simulink library "MantaFSController_cl"  (R2020a)
settings: Solver=VariableStepAuto  StartTime=0.0  StopTime=10.0  RelTol=1e-3
undefined symbols (not defined in the file or in its folder): a, env, FLIGHTCONTROLLER, fltCtrl, initializeBussesFromBlock, pthCtrl1, pthCtrl2, slfCtrl, thr, vhcl, wnch
libraries: simulink x21, angleBtw2Vecs_ul x9, pathGeometry_ul x6, filteredPIDController_ul x5, ctrlAllocMatrix_cl x4, tanFrameProjection_ul x4, vectorNormalizer_ul x4, velocityAngle_ul x4, filteredPIDControllerAWGS_ul x3, eulAng2RotMat_ul x3, vrlib x3, alphaBeta_ul x3
(part 1 of 3)
settings Model: Creator=jldanie5  LastModifiedBy=JohnJr
settings DataIOCC: ReturnWorkspaceOutputs=off
settings DebuggingCC: ArithmeticOperatorsInVariantConditions=warning
settings SFSimCC: CustomCodeUndefinedFunction=UseInterfaceOnly

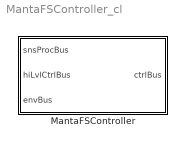
== system MantaFSController_cl ==
  MantaFSController : Subsystem  LoadFcn=initializeBussesFromBlock(gcb)  InitFcn=initializeBussesFromBlock(gcb)  StartFcn=initializeBussesFromBlock(gcb)  VariantControl=strcmpi(FLIGHTCONTROLLER,'MantaFSController')  mask{initPosForInitSStar=vhcl.initPosVecGnd.Value, fluidDensity=env.water.density.Value, LaRCtrl=fltCtrl, aeroStruct=vhcl.struct('OCT.aeroSurf'), LaRThr=thr.tether1, LaRWnch=wnch.winch1}
      mask prompts: initPosForInitSStar "Initial Position"; fluidDensity "Fluid Density"; LaRCtrl "Controller"; aeroStruct "Aerodynamic Structure"; LaRThr "Tether"; LaRWnch "Winch"
      settings: MinAlgLoopOccurrences=on
      mask DialogControl Container3 Prompt: Course Follow Params
      mask DialogControl Container4 Prompt: Setpoint To Output Params

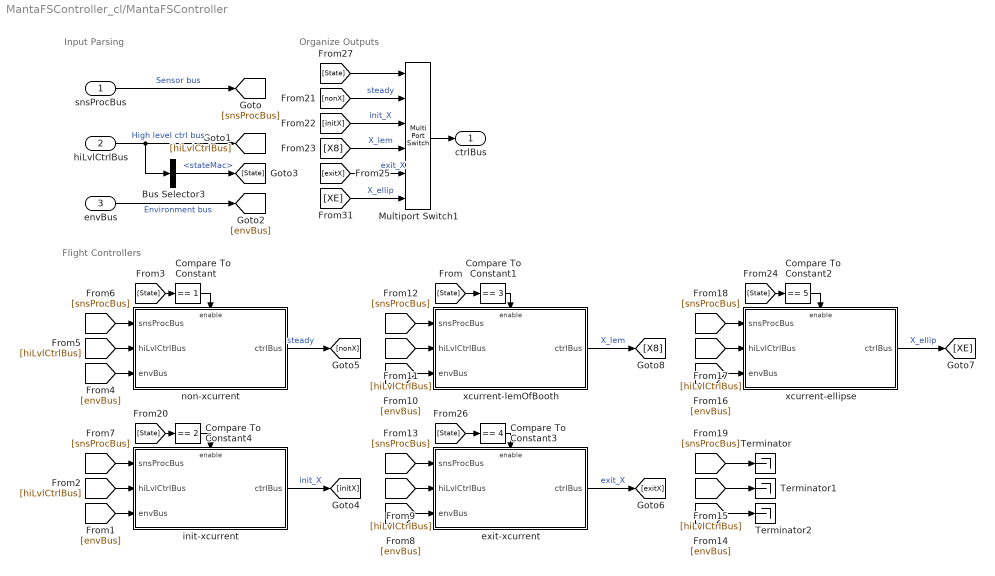
== system MantaFSController_cl/MantaFSController ==
  note: Organize Outputs
  note: Flight Controllers
  note: Input Parsing
  snsProcBus : Inport  OutDataTypeStr=Bus: sensorsProcessingBus
  hiLvlCtrlBus : Inport  Port=2  OutDataTypeStr=Bus: hiLvlCtrlBus
  envBus : Inport  Port=3  OutDataTypeStr=Bus: envBus
  Bus Selector3 : BusSelector  OutputSignals=stateMac
  Compare To Constant : simulink/Logic and Bit Operations/Compare To Constant  relop===  const=1  OutDataTypeStr=boolean
  Compare To Constant1 : simulink/Logic and Bit Operations/Compare To Constant  relop===  const=3  OutDataTypeStr=boolean
  Compare To Constant2 : simulink/Logic and Bit Operations/Compare To Constant  relop===  const=5  OutDataTypeStr=boolean
  Compare To Constant3 : simulink/Logic and Bit Operations/Compare To Constant  relop===  const=4  OutDataTypeStr=boolean
  Compare To Constant4 : simulink/Logic and Bit Operations/Compare To Constant  relop===  const=2  OutDataTypeStr=boolean
  Multiport Switch1 : MultiPortSwitch  Inputs=5  DataPortIndices={1,2,3,4,5,6}  DiagnosticForDefault=Warning
  Terminator : Terminator
  Terminator1 : Terminator
  Terminator2 : Terminator
  exit-xcurrent : Subsystem  TreatAsAtomicUnit=on
  init-xcurrent : Subsystem  TreatAsAtomicUnit=on
  non-xcurrent : Subsystem  TreatAsAtomicUnit=on
  xcurrent-ellipse : Subsystem  TreatAsAtomicUnit=on
  xcurrent-lemOfBooth : Subsystem  TreatAsAtomicUnit=on
  ctrlBus : Outport  OutDataTypeStr=Bus: fltCtrlBus  VectorParamsAs1DForOutWhenUnconnected=off
  wires:
  Bus Selector3/1 -> [State]  "<stateMac>"
  hiLvlCtrlBus/1 -> [hiLvlCtrlBus], Bus Selector3/1  "High level ctrl bus"
  snsProcBus/1 -> [snsProcBus]  "Sensor bus"
  envBus/1 -> [envBus]  "Environment bus"
  [X8] -> Multiport Switch1/4  "X_lem"
  Multiport Switch1/1 -> ctrlBus/1
  [State] -> Multiport Switch1/1
  [nonX] -> Multiport Switch1/2  "steady"
  [initX] -> Multiport Switch1/3  "init_X"
  [XE] -> Multiport Switch1/6  "X_ellip"
  [exitX] -> Multiport Switch1/5  "exit_X"
  [snsProcBus] -> init-xcurrent/1(snsProcBus)
  [hiLvlCtrlBus] -> init-xcurrent/2(hiLvlCtrlBus)
  [envBus] -> init-xcurrent/3(envBus)
  init-xcurrent/1(ctrlBus) -> [initX]  "init_X"
  non-xcurrent/1(ctrlBus) -> [nonX]  "steady"
  [envBus] -> non-xcurrent/3(envBus)
  [hiLvlCtrlBus] -> non-xcurrent/2(hiLvlCtrlBus)
  [snsProcBus] -> non-xcurrent/1(snsProcBus)
  xcurrent-lemOfBooth/1(ctrlBus) -> [X8]  "X_lem"
  [envBus] -> xcurrent-lemOfBooth/3(envBus)
  [hiLvlCtrlBus] -> xcurrent-lemOfBooth/2(hiLvlCtrlBus)
  [snsProcBus] -> xcurrent-lemOfBooth/1(snsProcBus)
  exit-xcurrent/1(ctrlBus) -> [exitX]  "exit_X"
  [envBus] -> exit-xcurrent/3(envBus)
  [hiLvlCtrlBus] -> exit-xcurrent/2(hiLvlCtrlBus)
  [snsProcBus] -> exit-xcurrent/1(snsProcBus)
  xcurrent-ellipse/1(ctrlBus) -> [XE]  "X_ellip"
  [envBus] -> xcurrent-ellipse/3(envBus)
  [hiLvlCtrlBus] -> xcurrent-ellipse/2(hiLvlCtrlBus)
  [snsProcBus] -> xcurrent-ellipse/1(snsProcBus)
  Compare To Constant/1 -> non-xcurrent/Enable
  [State] -> Compare To Constant/1
  [State] -> Compare To Constant1/1
  Compare To Constant1/1 -> xcurrent-lemOfBooth/Enable
  [State] -> Compare To Constant2/1
  Compare To Constant2/1 -> xcurrent-ellipse/Enable
  [State] -> Compare To Constant3/1
  Compare To Constant3/1 -> exit-xcurrent/Enable
  [State] -> Compare To Constant4/1
  Compare To Constant4/1 -> init-xcurrent/Enable
  [snsProcBus] -> Terminator/1
  [hiLvlCtrlBus] -> Terminator1/1
  [envBus] -> Terminator2/1

== system MantaFSController_cl/MantaFSController/exit-xcurrent ==
  snsProcBus : Inport  OutDataTypeStr=Bus: sensorsProcessingBus
  hiLvlCtrlBus : Inport  Port=2  OutDataTypeStr=Bus: hiLvlCtrlBus
  envBus : Inport  Port=3  OutDataTypeStr=Bus: envBus
  Enable : EnablePort
  Bus Creator : BusCreator  Inputs=5
  Bus Selector : BusSelector  OutputSignals=velocityVec,eulerAngles,angularVel
  Bus Selector1 : BusSelector  OutputSignals=vhclFlowVecs
  Constant4 : Constant  Value=zeros(3,1)
  Constant5 : Constant  Value=25
  Demux : Demux
  Ground{,1..3} (4 alike) : Ground
  Mux2 : Mux  Inputs=2
  Reshape{2,4,6..8} (5 alike) : Reshape  OutputDimensionality=Column vector (2-D)
  Selector : Selector  NumberOfDimensions=2  InputPortWidth=3  IndexOptions=Select all,Index vector (dialog)  Indices=[1 3],5  OutputSizes=1,1
  Terminator : Terminator
  Terminator5 : Terminator
  Vector Concatenate : Concatenate  NumInputs=4
  ctrlAllocation : ctrlAllocMatrix_cl/ctrlAllocMatrix  aeroStruct=aeroStruct  fluidDensity=fluidDensity
  pitchFlag1 : Constant  Value=pthCtrl1.RPMConst.Value
  ctrlBus : Outport  OutDataTypeStr=Bus: fltCtrlBus  VectorParamsAs1DForOutWhenUnconnected=off
  wires:
  [ctrlSurDefl] -> Bus Creator/1  "ctrlSurfDefl"
  Ground2/1 -> Bus Creator/3  "centralAngle"
  Ground/1 -> Bus Creator/2  "winchSpeeds"
  hiLvlCtrlBus/1 -> Terminator5/1
  Ground1/1 -> Bus Creator/4  "closestPathVariable"
  Bus Creator/1 -> ctrlBus/1
  [eul] -> ctrlAllocation/5
  [flowVecGnd] -> ctrlAllocation/3
  Bus Selector1/1 -> Selector/1  "<vhclFlowVecs>"
  Selector/1 -> Reshape2/1  "flowVelocityVec"
  Reshape7/1 -> [eul]
  Reshape8/1 -> [velGnd]
  Demux/2 -> Vector Concatenate/2
  Bus Selector/2 -> Reshape7/1  "<eulerAngles>"
  Bus Selector/1 -> Reshape8/1  "<velocityVec>"
  [angVel] -> ctrlAllocation/2
  Reshape2/1 -> [flowVecGnd]
  Vector Concatenate/1 -> Reshape4/1
  [velGnd] -> ctrlAllocation/1
  Constant4/1 -> ctrlAllocation/4
  Constant5/1 -> Vector Concatenate/3
  Bus Selector/3 -> Reshape6/1  "<angularVel>"
  envBus/1 -> Bus Selector1/1
  Demux/3 -> Terminator/1
  Demux/4 -> Vector Concatenate/4
  snsProcBus/1 -> Bus Selector/1
  ctrlAllocation/1 -> Demux/1
  Demux/1 -> Vector Concatenate/1
  Reshape6/1 -> [angVel]
  pitchFlag1/1 -> Mux2/2
  Ground3/1 -> Mux2/1  "turbOnOff"
  Mux2/1 -> Bus Creator/5  "turbOnOff"
  Reshape4/1 -> [ctrlSurDefl]

== system MantaFSController_cl/MantaFSController/init-xcurrent ==
  snsProcBus : Inport  OutDataTypeStr=Bus: sensorsProcessingBus
  hiLvlCtrlBus : Inport  Port=2  OutDataTypeStr=Bus: hiLvlCtrlBus
  envBus : Inport  Port=3  OutDataTypeStr=Bus: envBus
  Enable : EnablePort
  Bus Creator1 : BusCreator  Inputs=5
  Constant : Constant  Value=[0 0 -2 0]'
  Constant1 : Constant  Value=0
  Constant2 : Constant  Value=0
  Constant3 : Constant  Value=0
  Constant4 : Constant
  Mux2 : Mux  Inputs=2
  Reshape4 : Reshape  OutputDimensionality=Column vector (2-D)
  Terminator : Terminator
  Terminator1 : Terminator
  Terminator2 : Terminator
  pitchFlag1 : Constant  Value=pthCtrl1.RPMConst.Value
  ctrlBus : Outport  OutDataTypeStr=Bus: fltCtrlBus  VectorParamsAs1DForOutWhenUnconnected=off
  wires:
  envBus/1 -> Terminator1/1
  hiLvlCtrlBus/1 -> Terminator2/1
  snsProcBus/1 -> Terminator/1
  [turb] -> Bus Creator1/5  "turbOnOff"
  [sStar] -> Bus Creator1/4  "closestPathVariable"
  Constant3/1 -> [sStar]
  Constant1/1 -> [winchCmd]
  Constant2/1 -> [centralAngle]
  [centralAngle] -> Bus Creator1/3  "centralAngle"
  Bus Creator1/1 -> ctrlBus/1
  [ctrlSurDefl] -> Bus Creator1/1  "ctrlSurfDefl"
  [winchCmd] -> Bus Creator1/2  "winchSpeeds"
  pitchFlag1/1 -> Mux2/2
  Constant4/1 -> Mux2/1
  Mux2/1 -> [turb]  "turbOnOff"
  Constant/1 -> Reshape4/1
  Reshape4/1 -> [ctrlSurDefl]

== system MantaFSController_cl/MantaFSController/non-xcurrent ==
  snsProcBus : Inport  OutDataTypeStr=Bus: sensorsProcessingBus
  hiLvlCtrlBus : Inport  Port=2  OutDataTypeStr=Bus: hiLvlCtrlBus
  envBus : Inport  Port=3  OutDataTypeStr=Bus: envBus
  Enable : EnablePort
  LaRController : Subsystem  LoadFcn=initializeBussesFromBlock(gcb)  InitFcn=initializeBussesFromBlock(gcb)  StartFcn=initializeBussesFromBlock(gcb)  VariantControl=strcmpi(FLIGHTCONTROLLER,'LaRController')  mask{initPosForInitSStar=vhcl.initPosVecGnd.Value, fluidDensity=env.water.density.Value, LaRCtrl=slfCtrl, aeroStruct=vhcl.struct('OCT.aeroSurf'), LaRThr=thr.tether1, LaRWnch=wnch.winch1}
      mask prompts: initPosForInitSStar "Initial Position"; fluidDensity "Fluid Density"; LaRCtrl "Controller"; aeroStruct "Aerodynamic Structure"; LaRThr "Tether"; LaRWnch "Winch"
      settings: MinAlgLoopOccurrences=on
      mask DialogControl Container3 Prompt: courseFollow Params
      mask DialogControl Container4 Prompt: setpointToOutput Params
  ctrlBus : Outport  OutDataTypeStr=Bus: fltCtrlBus  VectorParamsAs1DForOutWhenUnconnected=off
  wires:
  snsProcBus/1 -> LaRController/1(snsProcBus)
  envBus/1 -> LaRController/3(envBus)
  hiLvlCtrlBus/1 -> LaRController/2(hiLvlCtrlBus)
  LaRController/1(ctrlBus) -> ctrlBus/1

== system MantaFSController_cl/MantaFSController/xcurrent-ellipse ==
  snsProcBus : Inport  OutDataTypeStr=Bus: sensorsProcessingBus
  hiLvlCtrlBus : Inport  Port=2  OutDataTypeStr=Bus: hiLvlCtrlBus
  envBus : Inport  Port=3  OutDataTypeStr=Bus: envBus
  Enable : EnablePort
  pathFollowingControllerManta1 : Subsystem  LoadFcn=initializeBussesFromBlock(gcb)  InitFcn=initializeBussesFromBlock(gcb)  StartFcn=initializeBussesFromBlock(gcb)  VariantControl=strcmpi(FLIGHTCONTROLLER,'pathFollowingControllerManta')  mask{initPosForInitSStar=vhcl.initPosVecGnd.Value, fluidDensity=env.water.density.Value, pathCtrl=pthCtrl2, aeroStruct=vhcl.struct('OCT.aeroSurf')}
      mask prompts: initPosForInitSStar "Initial Position"; fluidDensity "Fluid Density"; pathCtrl "Controller"; aeroStruct "Aerodynamic Structure"
      settings: MinAlgLoopOccurrences=on
      mask DialogControl Container3 Prompt: courseFollow Params
      mask DialogControl Container4 Prompt: setpointToOutput Params
  ctrlBus : Outport  OutDataTypeStr=Bus: fltCtrlBus  VectorParamsAs1DForOutWhenUnconnected=off
  wires:
  envBus/1 -> pathFollowingControllerManta1/3(envBus)
  hiLvlCtrlBus/1 -> pathFollowingControllerManta1/2(hiLvlCtrlBus)
  pathFollowingControllerManta1/1(ctrlBus) -> ctrlBus/1
  snsProcBus/1 -> pathFollowingControllerManta1/1(snsProcBus)

== system MantaFSController_cl/MantaFSController/xcurrent-lemOfBooth ==
  snsProcBus : Inport  OutDataTypeStr=Bus: sensorsProcessingBus
  hiLvlCtrlBus : Inport  Port=2  OutDataTypeStr=Bus: hiLvlCtrlBus
  envBus : Inport  Port=3  OutDataTypeStr=Bus: envBus
  Enable : EnablePort
  pathFollowingControllerManta : Subsystem  LoadFcn=initializeBussesFromBlock(gcb)  InitFcn=initializeBussesFromBlock(gcb)  StartFcn=initializeBussesFromBlock(gcb)  VariantControl=strcmpi(FLIGHTCONTROLLER,'pathFollowingControllerManta')  mask{initPosForInitSStar=vhcl.initPosVecGnd.Value, fluidDensity=env.water.density.Value, pathCtrl=pthCtrl1, aeroStruct=vhcl.struct('OCT.aeroSurf')}
      mask prompts: initPosForInitSStar "Initial Position"; fluidDensity "Fluid Density"; pathCtrl "Controller"; aeroStruct "Aerodynamic Structure"
      settings: MinAlgLoopOccurrences=on
      mask DialogControl Container3 Prompt: courseFollow Params
      mask DialogControl Container4 Prompt: setpointToOutput Params
  ctrlBus : Outport  OutDataTypeStr=Bus: fltCtrlBus  VectorParamsAs1DForOutWhenUnconnected=off
  wires:
  snsProcBus/1 -> pathFollowingControllerManta/1(snsProcBus)
  pathFollowingControllerManta/1(ctrlBus) -> ctrlBus/1
  hiLvlCtrlBus/1 -> pathFollowingControllerManta/2(hiLvlCtrlBus)
  envBus/1 -> pathFollowingControllerManta/3(envBus)

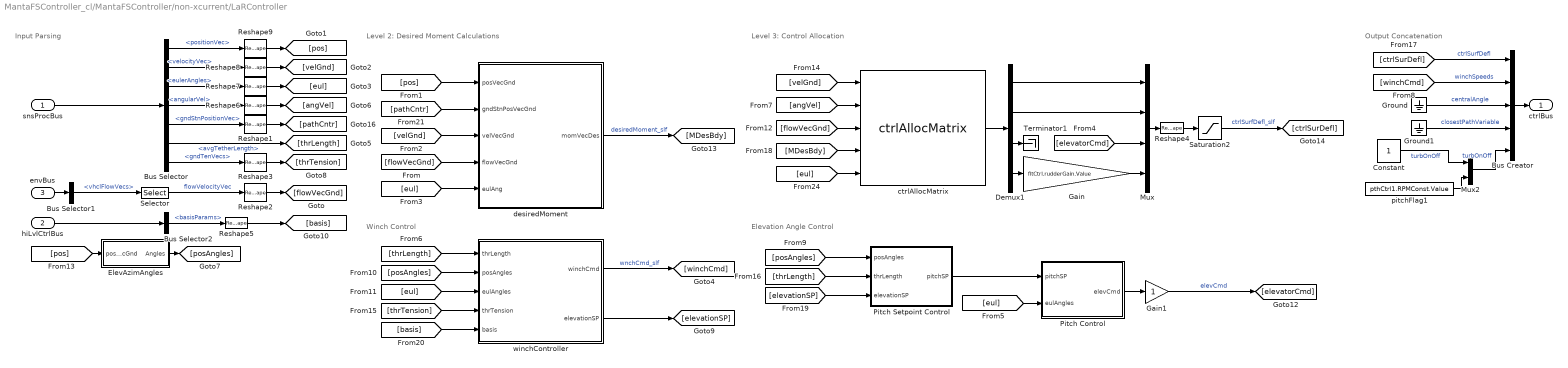
== system MantaFSController_cl/MantaFSController/non-xcurrent/LaRController ==
  note: Elevation Angle Control
  note: Input Parsing
  note: Level 2: Desired Moment Calculations
  note: Output Concatenation
  note: Level 3: Control Allocation
  note: Winch Control
  snsProcBus : Inport  OutDataTypeStr=Bus: sensorsProcessingBus
  hiLvlCtrlBus : Inport  Port=2  OutDataTypeStr=Bus: hiLvlCtrlBus
  envBus : Inport  Port=3  OutDataTypeStr=Bus: envBus
  Bus Creator : BusCreator  Inputs=5
  Bus Selector : BusSelector  OutputSignals=positionVec,velocityVec,eulerAngles,angularVel,gndStnPositionVec,avgTetherLength,gndTenVecs
  Bus Selector1 : BusSelector  OutputSignals=vhclFlowVecs
  Bus Selector2 : BusSelector  OutputSignals=basisParams
  Constant : Constant
  Demux1 : Demux
  ElevAzimAngles : Subsystem
  Gain : Gain  Gain=fltCtrl.rudderGain.Value
  Gain1 : Gain
  Ground : Ground
  Ground1 : Ground
  Mux : Mux
  Mux2 : Mux  Inputs=2
  Pitch Control : Subsystem
  Pitch Setpoint Control : Subsystem
  Reshape{1..9} (9 alike) : Reshape  OutputDimensionality=Column vector (2-D)
  Saturation2 : Saturate  UpperLimit=LaRCtrl.controlSigMax.upperLimit.Value  LowerLimit=LaRCtrl.controlSigMax.lowerLimit.Value
  Selector : Selector  NumberOfDimensions=2  InputPortWidth=3  IndexOptions=Select all,Index vector (dialog)  Indices=[1 3],5  OutputSizes=1,1
  Terminator1 : Terminator
  ctrlAllocMatrix : ctrlAllocMatrix_cl/ctrlAllocMatrix  aeroStruct=aeroStruct  fluidDensity=fluidDensity
  desiredMoment : Subsystem
  pitchFlag1 : Constant  Value=pthCtrl1.RPMConst.Value
  winchController : Subsystem  mask{thrC=LaRThr, ctrlC=LaRCtrl}
      mask prompts: thrC "Tether:"; ctrlC "Controller:"
  ctrlBus : Outport  OutDataTypeStr=Bus: fltCtrlBus  VectorParamsAs1DForOutWhenUnconnected=off
  wires:
  [elevationSP] -> Pitch Setpoint Control/3(elevationSP)
  winchController/2(elevationSP) -> [elevationSP]
  [thrLength] -> Pitch Setpoint Control/2(thrLength)
  Reshape3/1 -> [thrTension]
  [thrTension] -> winchController/4(thrTension)
  Bus Selector/7 -> Reshape3/1  "<gndTenVecs>"
  ElevAzimAngles/1(Angles) -> [posAngles]
  [pos] -> ElevAzimAngles/1(posVecGnd)
  [eul] -> winchController/3(eulAngles)
  [posAngles] -> winchController/2(posAngles)
  Gain1/1 -> [elevatorCmd]  "elevCmd"
  Pitch Setpoint Control/1(pitchSP) -> Pitch Control/1(pitchSP)
  [posAngles] -> Pitch Setpoint Control/1(posAngles)
  Pitch Control/1(elevCmd) -> Gain1/1
  [eul] -> Pitch Control/2(eulAngles)
  winchController/1(winchCmd) -> [winchCmd]  "wnchCmd_slf"
  [thrLength] -> winchController/1(thrLength)
  Bus Selector/6 -> [thrLength]  "<avgTetherLength>"
  [elevatorCmd] -> Mux/3
  Demux1/3 -> Terminator1/1
  Demux1/4 -> Gain/1
  Gain/1 -> Mux/4
  [flowVecGnd] -> desiredMoment/4(flowVecGnd)
  [eul] -> desiredMoment/5(eulAng)
  [velGnd] -> desiredMoment/3(velVecGnd)
  [pathCntr] -> desiredMoment/2(gndStnPosVecGnd)
  [pos] -> desiredMoment/1(posVecGnd)
  Bus Selector/5 -> Reshape1/1  "<gndStnPositionVec>"
  Reshape1/1 -> [pathCntr]
  Bus Selector1/1 -> Selector/1  "<vhclFlowVecs>"
  envBus/1 -> Bus Selector1/1
  Selector/1 -> Reshape2/1  "flowVelocityVec"
  [eul] -> ctrlAllocMatrix/5
  Reshape9/1 -> [pos]
  Reshape8/1 -> [velGnd]
  Reshape7/1 -> [eul]
  Reshape6/1 -> [angVel]
  Reshape2/1 -> [flowVecGnd]
  Saturation2/1 -> [ctrlSurDefl]  "ctrlSurfDefl_slf"
  [ctrlSurDefl] -> Bus Creator/1  "ctrlSurfDefl"
  [MDesBdy] -> ctrlAllocMatrix/4
  ctrlAllocMatrix/1 -> Demux1/1
  Demux1/2 -> Mux/2
  Demux1/1 -> Mux/1
  [flowVecGnd] -> ctrlAllocMatrix/3
  [velGnd] -> ctrlAllocMatrix/1
  [angVel] -> ctrlAllocMatrix/2
  Bus Selector/4 -> Reshape6/1  "<angularVel>"
  desiredMoment/1(momVecDes) -> [MDesBdy]  "desiredMoment_slf"
  Ground1/1 -> Bus Creator/4  "closestPathVariable"
  Ground/1 -> Bus Creator/3  "centralAngle"
  [winchCmd] -> Bus Creator/2  "winchSpeeds"
  Bus Creator/1 -> ctrlBus/1
  Bus Selector/3 -> Reshape7/1  "<eulerAngles>"
  Bus Selector/1 -> Reshape9/1  "<positionVec>"
  Bus Selector/2 -> Reshape8/1  "<velocityVec>"
  snsProcBus/1 -> Bus Selector/1
  pitchFlag1/1 -> Mux2/2
  Constant/1 -> Mux2/1  "turbOnOff"
  Mux2/1 -> Bus Creator/5  "turbOnOff"
  Mux/1 -> Reshape4/1
  Reshape4/1 -> Saturation2/1
  Bus Selector2/1 -> Reshape5/1  "<basisParams>"
  hiLvlCtrlBus/1 -> Bus Selector2/1
  Reshape5/1 -> [basis]
  [basis] -> winchController/5(basis)

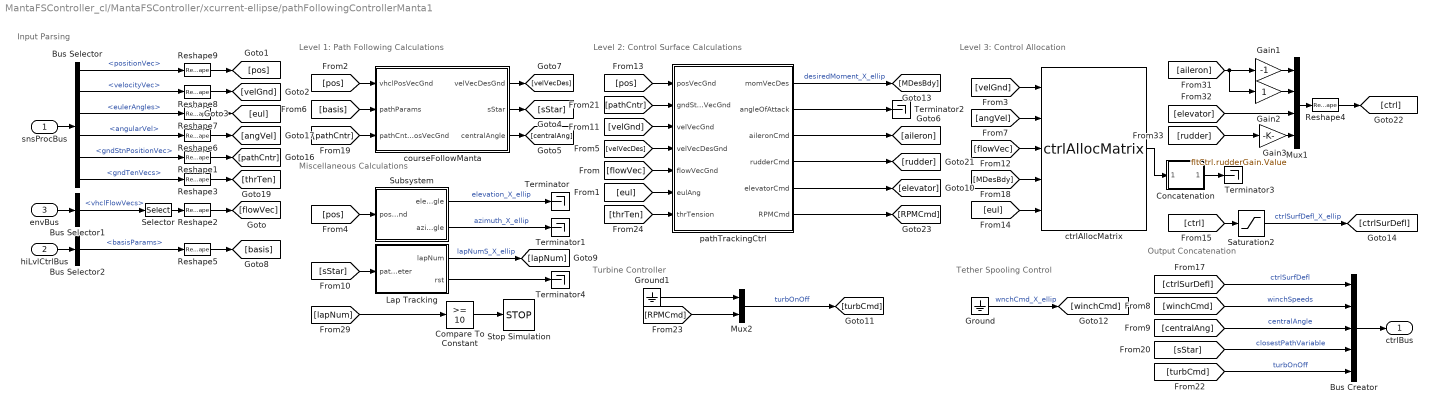
== system MantaFSController_cl/MantaFSController/xcurrent-ellipse/pathFollowingControllerManta1 ==
  note: Turbine Controller
  note: Input Parsing
  note: Level 1: Path Following Calculations
  note: Level 2: Control Surface Calculations
  note: Tether Spooling Control
  note: Output Concatenation
  note: Level 3: Control Allocation
  note: Miscellaneous Calculations
  snsProcBus : Inport  OutDataTypeStr=Bus: sensorsProcessingBus
  hiLvlCtrlBus : Inport  Port=2  OutDataTypeStr=Bus: hiLvlCtrlBus
  envBus : Inport  Port=3  OutDataTypeStr=Bus: envBus
  Bus Creator : BusCreator  Inputs=5
  Bus Selector : BusSelector  OutputSignals=positionVec,velocityVec,eulerAngles,angularVel,gndStnPositionVec,gndTenVecs
  Bus Selector1 : BusSelector  OutputSignals=vhclFlowVecs
  Bus Selector2 : BusSelector  OutputSignals=basisParams
  Compare To Constant : simulink/Logic and Bit Operations/Compare To Constant  relop=>=  const=10  OutDataTypeStr=boolean
  Concatenation : Subsystem
  Gain1 : Gain  Gain=-1
  Gain2 : Gain
  Gain3 : Gain  Gain=fltCtrl.rudderGain.Value
  Ground : Ground
  Ground1 : Ground
  Lap Tracking : Subsystem
  Mux1 : Mux
  Mux2 : Mux  Inputs=2
  Reshape{1..9} (9 alike) : Reshape  OutputDimensionality=Column vector (2-D)
  Saturation2 : Saturate  UpperLimit=pathCtrl.controlSigMax.upperLimit.Value  LowerLimit=pathCtrl.controlSigMax.lowerLimit.Value
  Selector : Selector  NumberOfDimensions=2  InputPortWidth=3  IndexOptions=Select all,Index vector (dialog)  Indices=[1 3],5  OutputSizes=1,1
  Stop Simulation : Stop
  Subsystem : Subsystem
  Terminator{,1..4} (5 alike) : Terminator
  courseFollowManta : Subsystem
  ctrlAllocMatrix : ctrlAllocMatrix_cl/ctrlAllocMatrix  aeroStruct=aeroStruct  fluidDensity=fluidDensity
  pathTrackingCtrl : Subsystem
  ctrlBus : Outport  OutDataTypeStr=Bus: fltCtrlBus  VectorParamsAs1DForOutWhenUnconnected=off
  wires:
  [thrTen] -> pathTrackingCtrl/7(thrTension)
  [ctrl] -> Saturation2/1
  pathTrackingCtrl/4(rudderCmd) -> [rudder]
  pathTrackingCtrl/2(angleOfAttack) -> Terminator2/1
  pathTrackingCtrl/3(aileronCmd) -> [aileron]
  Gain2/1 -> Mux1/2
  Gain3/1 -> Mux1/4
  [aileron] -> Gain2/1, Gain1/1
  [rudder] -> Gain3/1
  [elevator] -> Mux1/3
  Gain1/1 -> Mux1/1
  Compare To Constant/1 -> Stop Simulation/1
  [lapNum] -> Compare To Constant/1
  Ground/1 -> [winchCmd]  "wnchCmd_X_ellip"
  Lap Tracking/1(lapNum) -> [lapNum]  "lapNumS_X_ellip"
  Lap Tracking/2(rst) -> Terminator4/1
  [sStar] -> Lap Tracking/1(pathParameter)
  Subsystem/2(azimuth Angle) -> Terminator1/1  "azimuth_X_ellip"
  Subsystem/1(elevationAngle) -> Terminator/1  "elevation_X_ellip"
  [pos] -> Subsystem/1(posVecGnd)
  [basis] -> courseFollowManta/2(pathParams)
  [flowVec] -> pathTrackingCtrl/5(flowVecGnd)
  [eul] -> pathTrackingCtrl/6(eulAng)
  [velVecDes] -> pathTrackingCtrl/4(velVecDesGnd)
  [velGnd] -> pathTrackingCtrl/3(velVecGnd)
  [pathCntr] -> pathTrackingCtrl/2(gndStnPosVecGnd)
  [pos] -> pathTrackingCtrl/1(posVecGnd)
  [pathCntr] -> courseFollowManta/3(pathCntrPosVecGnd)
  Bus Selector/5 -> Reshape1/1  "<gndStnPositionVec>"
  Reshape1/1 -> [pathCntr]
  Bus Selector1/1 -> Selector/1  "<vhclFlowVecs>"
  envBus/1 -> Bus Selector1/1
  Selector/1 -> Reshape2/1
  [eul] -> ctrlAllocMatrix/5
  Reshape9/1 -> [pos]
  Reshape8/1 -> [velGnd]
  Reshape7/1 -> [eul]
  Reshape6/1 -> [angVel]
  Reshape2/1 -> [flowVec]
  Saturation2/1 -> [ctrlSurDefl]  "ctrlSurfDefl_X_ellip"
  Reshape5/1 -> [basis]
  Bus Selector2/1 -> Reshape5/1  "<basisParams>"
  [ctrlSurDefl] -> Bus Creator/1  "ctrlSurfDefl"
  [MDesBdy] -> ctrlAllocMatrix/4
  [flowVec] -> ctrlAllocMatrix/3
  [velGnd] -> ctrlAllocMatrix/1
  [angVel] -> ctrlAllocMatrix/2
  Bus Selector/4 -> Reshape6/1  "<angularVel>"
  pathTrackingCtrl/1(momVecDes) -> [MDesBdy]  "desiredMoment_X_ellip"
  courseFollowManta/3(centralAngle) -> [centralAng]
  [sStar] -> Bus Creator/4  "closestPathVariable"
  [centralAng] -> Bus Creator/3  "centralAngle"
  hiLvlCtrlBus/1 -> Bus Selector2/1
  courseFollowManta/2(sStar) -> [sStar]
  [winchCmd] -> Bus Creator/2  "winchSpeeds"
  Bus Creator/1 -> ctrlBus/1
  [pos] -> courseFollowManta/1("vhclPosVecGnd ")
  Bus Selector/3 -> Reshape7/1  "<eulerAngles>"
  Bus Selector/1 -> Reshape9/1  "<positionVec>"
  Bus Selector/2 -> Reshape8/1  "<velocityVec>"
  snsProcBus/1 -> Bus Selector/1
  courseFollowManta/1(velVecDesGnd) -> [velVecDes]
  Reshape3/1 -> [thrTen]
  Bus Selector/6 -> Reshape3/1  "<gndTenVecs>"
  pathTrackingCtrl/5(elevatorCmd) -> [elevator]
  pathTrackingCtrl/6(RPMCmd) -> [RPMCmd]
  Mux2/1 -> [turbCmd]  "turbOnOff"
  Ground1/1 -> Mux2/1
  [RPMCmd] -> Mux2/2
  [turbCmd] -> Bus Creator/5  "turbOnOff"
  ctrlAllocMatrix/1 -> Concatenation/1(In1)
  Concatenation/1(Out1) -> Terminator3/1
  Mux1/1 -> Reshape4/1
  Reshape4/1 -> [ctrl]

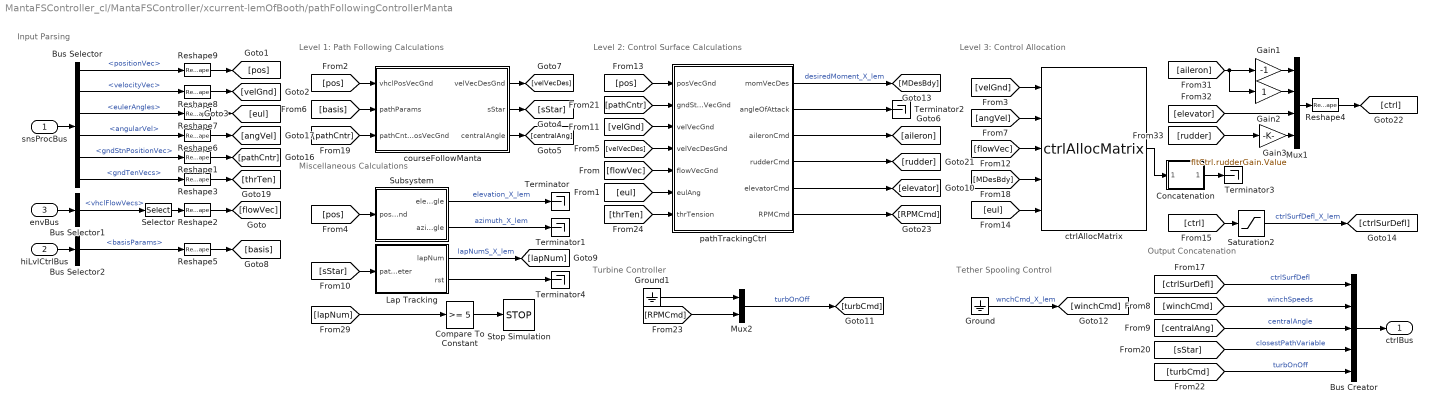
== system MantaFSController_cl/MantaFSController/xcurrent-lemOfBooth/pathFollowingControllerManta ==
  note: Turbine Controller
  note: Input Parsing
  note: Level 1: Path Following Calculations
  note: Level 2: Control Surface Calculations
  note: Tether Spooling Control
  note: Output Concatenation
  note: Level 3: Control Allocation
  note: Miscellaneous Calculations
  snsProcBus : Inport  OutDataTypeStr=Bus: sensorsProcessingBus
  hiLvlCtrlBus : Inport  Port=2  OutDataTypeStr=Bus: hiLvlCtrlBus
  envBus : Inport  Port=3  OutDataTypeStr=Bus: envBus
  Bus Creator : BusCreator  Inputs=5
  Bus Selector : BusSelector  OutputSignals=positionVec,velocityVec,eulerAngles,angularVel,gndStnPositionVec,gndTenVecs
  Bus Selector1 : BusSelector  OutputSignals=vhclFlowVecs
  Bus Selector2 : BusSelector  OutputSignals=basisParams
  Compare To Constant : simulink/Logic and Bit Operations/Compare To Constant  relop=>=  const=5  OutDataTypeStr=boolean
  Concatenation : Subsystem
  Gain1 : Gain  Gain=-1
  Gain2 : Gain
  Gain3 : Gain  Gain=fltCtrl.rudderGain.Value
  Ground : Ground
  Ground1 : Ground
  Lap Tracking : Subsystem
  Mux1 : Mux
  Mux2 : Mux  Inputs=2
  Reshape{1..9} (9 alike) : Reshape  OutputDimensionality=Column vector (2-D)
  Saturation2 : Saturate  UpperLimit=pathCtrl.controlSigMax.upperLimit.Value  LowerLimit=pathCtrl.controlSigMax.lowerLimit.Value
  Selector : Selector  NumberOfDimensions=2  InputPortWidth=3  IndexOptions=Select all,Index vector (dialog)  Indices=[1 3],5  OutputSizes=1,1
  Stop Simulation : Stop
  Subsystem : Subsystem
  Terminator{,1..4} (5 alike) : Terminator
  courseFollowManta : Subsystem
  ctrlAllocMatrix : ctrlAllocMatrix_cl/ctrlAllocMatrix  aeroStruct=aeroStruct  fluidDensity=fluidDensity
  pathTrackingCtrl : Subsystem
  ctrlBus : Outport  OutDataTypeStr=Bus: fltCtrlBus  VectorParamsAs1DForOutWhenUnconnected=off
  wires:
  [thrTen] -> pathTrackingCtrl/7(thrTension)
  [ctrl] -> Saturation2/1
  pathTrackingCtrl/4(rudderCmd) -> [rudder]
  pathTrackingCtrl/2(angleOfAttack) -> Terminator2/1
  pathTrackingCtrl/3(aileronCmd) -> [aileron]
  Gain2/1 -> Mux1/2
  Gain3/1 -> Mux1/4
  [aileron] -> Gain2/1, Gain1/1
  [rudder] -> Gain3/1
  [elevator] -> Mux1/3
  Gain1/1 -> Mux1/1
  Compare To Constant/1 -> Stop Simulation/1
  [lapNum] -> Compare To Constant/1
  Ground/1 -> [winchCmd]  "wnchCmd_X_lem"
  Lap Tracking/1(lapNum) -> [lapNum]  "lapNumS_X_lem"
  Lap Tracking/2(rst) -> Terminator4/1
  [sStar] -> Lap Tracking/1(pathParameter)
  Subsystem/2(azimuth Angle) -> Terminator1/1  "azimuth_X_lem"
  Subsystem/1(elevationAngle) -> Terminator/1  "elevation_X_lem"
  [pos] -> Subsystem/1(posVecGnd)
  [basis] -> courseFollowManta/2(pathParams)
  [flowVec] -> pathTrackingCtrl/5(flowVecGnd)
  [eul] -> pathTrackingCtrl/6(eulAng)
  [velVecDes] -> pathTrackingCtrl/4(velVecDesGnd)
  [velGnd] -> pathTrackingCtrl/3(velVecGnd)
  [pathCntr] -> pathTrackingCtrl/2(gndStnPosVecGnd)
  [pos] -> pathTrackingCtrl/1(posVecGnd)
  [pathCntr] -> courseFollowManta/3(pathCntrPosVecGnd)
  Bus Selector/5 -> Reshape1/1  "<gndStnPositionVec>"
  Reshape1/1 -> [pathCntr]
  Bus Selector1/1 -> Selector/1  "<vhclFlowVecs>"
  envBus/1 -> Bus Selector1/1
  Selector/1 -> Reshape2/1
  [eul] -> ctrlAllocMatrix/5
  Reshape9/1 -> [pos]
  Reshape8/1 -> [velGnd]
  Reshape7/1 -> [eul]
  Reshape6/1 -> [angVel]
  Reshape2/1 -> [flowVec]
  Saturation2/1 -> [ctrlSurDefl]  "ctrlSurfDefl_X_lem"
  Reshape5/1 -> [basis]
  Bus Selector2/1 -> Reshape5/1  "<basisParams>"
  [ctrlSurDefl] -> Bus Creator/1  "ctrlSurfDefl"
  [MDesBdy] -> ctrlAllocMatrix/4
  [flowVec] -> ctrlAllocMatrix/3
  [velGnd] -> ctrlAllocMatrix/1
  [angVel] -> ctrlAllocMatrix/2
  Bus Selector/4 -> Reshape6/1  "<angularVel>"
  pathTrackingCtrl/1(momVecDes) -> [MDesBdy]  "desiredMoment_X_lem"
  courseFollowManta/3(centralAngle) -> [centralAng]
  [sStar] -> Bus Creator/4  "closestPathVariable"
  [centralAng] -> Bus Creator/3  "centralAngle"
  hiLvlCtrlBus/1 -> Bus Selector2/1
  courseFollowManta/2(sStar) -> [sStar]
  [winchCmd] -> Bus Creator/2  "winchSpeeds"
  Bus Creator/1 -> ctrlBus/1
  [pos] -> courseFollowManta/1("vhclPosVecGnd ")
  Bus Selector/3 -> Reshape7/1  "<eulerAngles>"
  Bus Selector/1 -> Reshape9/1  "<positionVec>"
  Bus Selector/2 -> Reshape8/1  "<velocityVec>"
  snsProcBus/1 -> Bus Selector/1
  courseFollowManta/1(velVecDesGnd) -> [velVecDes]
  Reshape3/1 -> [thrTen]
  Bus Selector/6 -> Reshape3/1  "<gndTenVecs>"
  pathTrackingCtrl/5(elevatorCmd) -> [elevator]
  pathTrackingCtrl/6(RPMCmd) -> [RPMCmd]
  Mux2/1 -> [turbCmd]  "turbOnOff"
  Ground1/1 -> Mux2/1
  [RPMCmd] -> Mux2/2
  [turbCmd] -> Bus Creator/5  "turbOnOff"
  ctrlAllocMatrix/1 -> Concatenation/1(In1)
  Concatenation/1(Out1) -> Terminator3/1
  Mux1/1 -> Reshape4/1
  Reshape4/1 -> [ctrl]

== system MantaFSController_cl/MantaFSController/non-xcurrent/LaRController/ElevAzimAngles ==
  posVecGnd : Inport
  Atan1 : Trigonometry  Operator=atan2
  Atan2 : Trigonometry  Operator=atan2
  Gain : Gain  Gain=180/pi
  Gain1 : Gain  Gain=180/pi
  Mux : Mux  Inputs=2
  Selector1 : Selector  InputPortWidth=3  IndexOptions=Index vector (dialog)  Indices=1  OutputSizes=1
  Selector2 : Selector  InputPortWidth=3  IndexOptions=Index vector (dialog)  Indices=[1 2]  OutputSizes=1
  Selector3 : Selector  InputPortWidth=3  IndexOptions=Index vector (dialog)  Indices=3  OutputSizes=1
  Selector4 : Selector  InputPortWidth=3  IndexOptions=Index vector (dialog)  Indices=2  OutputSizes=1
  Sqrt1 : Sqrt  SaturateOnIntegerOverflow=on
  Sqrt2 : Sqrt  SaturateOnIntegerOverflow=on
  Square1 : Math  Operator=square  SignedPower=on  SaturateOnIntegerOverflow=on
  Square2 : Math  Operator=square  SignedPower=on  SaturateOnIntegerOverflow=on
  Sum of Elements : Sum  Inputs=+
  Sum of Elements1 : Sum  Inputs=+
  Angles : Outport
  wires:
  Mux/1 -> Angles/1
  Gain1/1 -> Mux/2  "azimuth_slf"
  Gain/1 -> Mux/1  "elevation_slf"
  Square2/1 -> Sum of Elements1/1
  Sqrt2/1 -> Atan2/2
  Atan2/1 -> Gain1/1
  posVecGnd/1 -> Selector2/1, Selector1/1, Selector4/1, Selector3/1
  Sum of Elements1/1 -> Sqrt2/1
  Selector1/1 -> Square2/1
  Selector4/1 -> Atan2/1
  Selector2/1 -> Square1/1
  Atan1/1 -> Gain/1
  Sum of Elements/1 -> Sqrt1/1
  Selector3/1 -> Atan1/1
  Square1/1 -> Sum of Elements/1
  Sqrt1/1 -> Atan1/2

== system MantaFSController_cl/MantaFSController/non-xcurrent/LaRController/Pitch Control ==
  pitchSP : Inport
  eulAngles : Inport  Port=2
  Add1 : Sum  Inputs=-+
  Gain2 : Gain  Gain=pi/180
  Selector2 : Selector  InputPortWidth=3  IndexOptions=Index vector (dialog)  Indices=2  OutputSizes=1
  filteredPIDControllerAW : filteredPIDControllerAW_ul/filteredPIDControllerAW  kp=LaRCtrl.elevCmd.kp.Value  ki=LaRCtrl.elevCmd.ki.Value  kd=LaRCtrl.elevCmd.kd.Value  tau=LaRCtrl.elevCmd.tau.Value  cmax=LaRCtrl.controlSigMax.upperLimit.Value  cmin=LaRCtrl.controlSigMax.lowerLimit.Value
  elevCmd : Outport
  wires:
  Add1/1 -> filteredPIDControllerAW/1  "err"
  Gain2/1 -> Add1/1
  eulAngles/1 -> Selector2/1
  pitchSP/1 -> Gain2/1
  filteredPIDControllerAW/1 -> elevCmd/1  "elevCmd"
  Selector2/1 -> Add1/2  "pitch"

== system MantaFSController_cl/MantaFSController/non-xcurrent/LaRController/Pitch Setpoint Control ==
  posAngles : Inport
  thrLength : Inport  Port=2
  elevationSP : Inport  Port=3
  1-D Lookup Table : Lookup_n-D  NumberOfTableDimensions=1  BreakpointsForDimension1=LaRCtrl.pitchTime.Value  Table=LaRCtrl.pitchLookup.Value  InterpMethod=Flat  InternalRulePriority=Speed  RndMeth=Simplest  InputSameDT=on
  Clock : Clock
  Constant5 : Constant  Value=LaRCtrl.pitchSP.kd.Value
  Constant6 : Constant  Value=LaRCtrl.pitchSP.tau.Value
  Gain : Gain
  Multiport Switch : MultiPortSwitch  DataPortOrder=Specify indices  Inputs=2  DataPortIndices={0,1,2}
  Mux : Mux
  Polynomial1 : Polyval  Coefs=[LaRCtrl.pitchSPkpSlope.Value LaRCtrl.pitchSPkpInt.Value]
  Polynomial2 : Polyval  Coefs=[LaRCtrl.pitchSPkiSlope.Value LaRCtrl.pitchSPkiInt.Value]
  Saturation : Saturate  UpperLimit=LaRCtrl.pitchAngleMax.upperLimit.Value  LowerLimit=LaRCtrl.pitchAngleMax.lowerLimit.Value
  Selector : Selector  InputPortWidth=2  IndexOptions=Index vector (dialog)  Indices=1  OutputSizes=1
  Subtract : Sum  Inputs=+-
  Terminator2 : Terminator
  filteredPIDControllerAWGS : filteredPIDControllerAWGS_ul/filteredPIDControllerAWGS  cmax=LaRCtrl.pitchAngleMax.upperLimit.Value  cmin=LaRCtrl.pitchAngleMax.lowerLimit.Value
  pitchDes : Constant  Value=LaRCtrl.pitchConst.Value
  pitchFlag : Constant  Value=LaRCtrl.pitchCtrl.Value
  pitchSP : Outport
  wires:
  Saturation/1 -> Multiport Switch/4
  filteredPIDControllerAWGS/1 -> Saturation/1
  thrLength/1 -> Polynomial1/1, Polynomial2/1
  Mux/1 -> [gains]
  [gains] -> filteredPIDControllerAWGS/2
  Constant6/1 -> Mux/4  "tau"
  Constant5/1 -> Mux/3  "kd"
  Polynomial2/1 -> Mux/2  "ki"
  Polynomial1/1 -> Mux/1  "kp"
  Subtract/1 -> filteredPIDControllerAWGS/1
  elevationSP/1 -> Terminator2/1, Gain/1
  1-D Lookup Table/1 -> Multiport Switch/3
  Gain/1 -> Subtract/1  "elevationSP"
  Selector/1 -> Subtract/2  "elevationAngle"
  Clock/1 -> 1-D Lookup Table/1
  posAngles/1 -> Selector/1
  pitchDes/1 -> Multiport Switch/2
  Multiport Switch/1 -> pitchSP/1  "pitchSP"
  pitchFlag/1 -> Multiport Switch/1

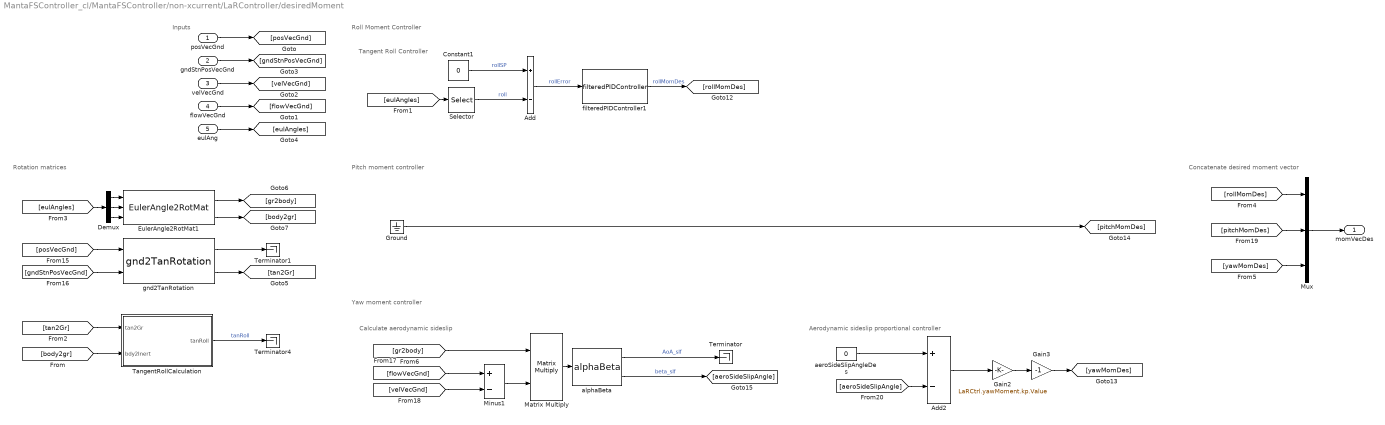
== system MantaFSController_cl/MantaFSController/non-xcurrent/LaRController/desiredMoment ==
  note: Roll Moment Controller
  note: Pitch moment controller
  note: Yaw moment controller
  note: Calculate aerodynamic sideslip
  note: Aerodynamic sideslip proportional controller
  note: Concatenate desired moment vector
  note: Tangent Roll Controller
  note: Rotation matrices
  note: Inputs
  posVecGnd : Inport
  gndStnPosVecGnd : Inport  Port=2
  velVecGnd : Inport  Port=3
  flowVecGnd : Inport  Port=4
  eulAng : Inport  Port=5
  Add : Sum  Inputs=+-
  Add2 : Sum  Inputs=+-
  Constant1 : Constant  Value=0
  Demux : Demux  Outputs=3
  EulerAngle2RotMat1 : eulAng2RotMat_ul/EulerAngle2RotMat  SystemSampleTime=-1  Latency=0  AutoFrameSizeCalculation=off
  Gain2 : Gain  Gain=LaRCtrl.yawMoment.kp.Value
  Gain3 : Gain  Gain=-1
  Ground : Ground
  Matrix Multiply : Product  Multiplication=Matrix(*)
  Minus1 : Sum  Inputs=+-
  Mux : Mux  Inputs=3
  Selector : Selector  InputPortWidth=3  IndexOptions=Index vector (dialog)  Indices=1  OutputSizes=1
  TangentRollCalculation : Subsystem
  Terminator : Terminator
  Terminator1 : Terminator
  Terminator4 : Terminator
  aeroSideSlipAngleDes : Constant  Value=0
  alphaBeta : alphaBeta_ul/alphaBeta  SystemSampleTime=-1  Latency=0  AutoFrameSizeCalculation=off
  filteredPIDController1 : filteredPIDController_ul/filteredPIDController  kp=LaRCtrl.rollMoment.kp.Value  ki=LaRCtrl.rollMoment.ki.Value  kd=LaRCtrl.rollMoment.kd.Value  Value=LaRCtrl.rollMoment.tau.Value  externalReset=none
  gnd2TanRotation : gnd2TanRotation_ul/gnd2TanRotation  SystemSampleTime=-1  Latency=0  AutoFrameSizeCalculation=off
  momVecDes : Outport  VectorParamsAs1DForOutWhenUnconnected=off
  wires:
  [body2gr] -> TangentRollCalculation/2(bdy2Inert)
  [tan2Gr] -> TangentRollCalculation/1(tan2Gr)
  TangentRollCalculation/1(tanRoll) -> Terminator4/1  "tanRoll"
  Ground/1 -> [pitchMomDes]
  Selector/1 -> Add/2  "roll"
  [eulAngles] -> Selector/1
  [eulAngles] -> Demux/1
  eulAng/1 -> [eulAngles]
  posVecGnd/1 -> [posVecGnd]
  velVecGnd/1 -> [velVecGnd]
  Add/1 -> filteredPIDController1/1  "rollError"
  flowVecGnd/1 -> [flowVecGnd]
  filteredPIDController1/1 -> [rollMomDes]  "rollMomDes"
  Gain2/1 -> Gain3/1
  Minus1/1 -> Matrix Multiply/2
  [velVecGnd] -> Minus1/2
  [flowVecGnd] -> Minus1/1
  Demux/3 -> EulerAngle2RotMat1/3
  Demux/1 -> EulerAngle2RotMat1/1
  Demux/2 -> EulerAngle2RotMat1/2
  EulerAngle2RotMat1/2 -> [body2gr]
  EulerAngle2RotMat1/1 -> [gr2body]
  [gr2body] -> Matrix Multiply/1
  Matrix Multiply/1 -> alphaBeta/1
  Add2/1 -> Gain2/1
  aeroSideSlipAngleDes/1 -> Add2/1
  Mux/1 -> momVecDes/1
  Gain3/1 -> [yawMomDes]
  [pitchMomDes] -> Mux/2
  gndStnPosVecGnd/1 -> [gndStnPosVecGnd]
  Constant1/1 -> Add/1  "rollSP"
  [posVecGnd] -> gnd2TanRotation/1
  [gndStnPosVecGnd] -> gnd2TanRotation/2
  gnd2TanRotation/2 -> [tan2Gr]
  gnd2TanRotation/1 -> Terminator1/1
  [rollMomDes] -> Mux/1
  [yawMomDes] -> Mux/3
  [aeroSideSlipAngle] -> Add2/2
  alphaBeta/1 -> Terminator/1  "AoA_slf"
  alphaBeta/2 -> [aeroSideSlipAngle]  "beta_slf"

== system MantaFSController_cl/MantaFSController/non-xcurrent/LaRController/winchController ==
  thrLength : Inport
  posAngles : Inport  Port=2
  eulAngles : Inport  Port=3
  thrTension : Inport  Port=4
  basis : Inport  Port=5
  Constant : Constant  Value=LaRCtrl.LaRelevationSP.Value
  Constant1 : Constant  Value=LaRCtrl.winchActive.Value
  Constant2 : Constant  Value=LaRCtrl.LaRelevationSP.Value
  Gain : Gain  Gain=180/pi
  Ground : Ground
  MATLAB Function : MATLAB Function  TreatAsAtomicUnit=on  mask{leash=LaRCtrl.shortLeashLength.Value, spd=LaRCtrl.nomSpoolSpeed.Value, coneWidth=LaRCtrl.LaRelevationSPErr.Value}
      mask prompts: leash "Short Leash Length [m]"; spd "Nominal Spool Speed [m/s]"; coneWidth "Elevation Angle Error Threshold"
  MATLAB Function1 : MATLAB Function  TreatAsAtomicUnit=on  mask{elevSP1=LaRCtrl.LaRelevationSP.Value, elevSP2=50}
      mask prompts: elevSP1 "Nominal Elevation Setpoint [deg]"; elevSP2 "Final Elevation Setpoint [deg]"
  Selector : Selector  InputPortWidth=5  IndexOptions=Index vector (dialog)  Indices=3  OutputSizes=1
  Switch : Switch  Criteria=u2 > Threshold  Threshold=.5
  Terminator : Terminator
  Terminator1 : Terminator
  winchCmd : Outport
  elevationSP : Outport  Port=2
  wires:
  MATLAB Function1/1(elevationSP) -> Terminator/1
  Constant/1 -> MATLAB Function/5(elevSP)
  [thrLength] -> MATLAB Function1/1(thrLength)
  [thrTension] -> MATLAB Function/2(thrTension)
  thrTension/1 -> [thrTension]
  [thrLength] -> MATLAB Function/1(thrLength)
  [posAngles] -> MATLAB Function/3(posAng)
  [eul] -> MATLAB Function/4(eulAng)
  eulAngles/1 -> [eul]
  [winchCmd] -> winchCmd/1
  posAngles/1 -> [posAngles]
  thrLength/1 -> [thrLength]
  Switch/1 -> [winchCmd]
  MATLAB Function/1(Ctrl) -> Switch/1
  Constant1/1 -> Switch/2
  Ground/1 -> Switch/3
  basis/1 -> Selector/1
  Selector/1 -> [elevSP]
  [elevSP] -> Gain/1
  Constant2/1 -> Terminator1/1
  Gain/1 -> elevationSP/1

== system MantaFSController_cl/MantaFSController/xcurrent-ellipse/pathFollowingControllerManta1/Concatenation ==
  In1 : Inport
  Demux1 : Demux
  Gain : Gain  Gain=pathCtrl.rudderGain.Value
  Mux : Mux
  Out1 : Outport
  wires:
  In1/1 -> Demux1/1
  Mux/1 -> Out1/1
  Demux1/4 -> Gain/1
  Gain/1 -> Mux/4  "rudderCmd"
  Demux1/2 -> Mux/2  "starBrdCmd"
  Demux1/1 -> Mux/1  "portCmd"
  Demux1/3 -> Mux/3  "elevCmd"

== system MantaFSController_cl/MantaFSController/xcurrent-ellipse/pathFollowingControllerManta1/Lap Tracking ==
  pathParameter : Inport
  Add2 : Sum
  Compare To Constant1 : simulink/Logic and Bit Operations/Compare To Constant  relop=>=  const=10  OutDataTypeStr=boolean
  Compare To Constant3 : simulink/Logic and Bit Operations/Compare To Constant  relop=<=  const=0.1  OutDataTypeStr=boolean
  Compare To Constant4 : simulink/Logic and Bit Operations/Compare To Constant  relop=>=  const=0.9  OutDataTypeStr=boolean
  Data Type Conversion2 : DataTypeConversion  OutDataTypeStr=double
  Logical Operator1 : Logic  Inputs=4  AllPortsSameDT=off  OutDataTypeStr=boolean
  Memory : Memory  InitialCondition=false
  Memory3 : Memory
  Memory4 : Memory
  Subsystem : Subsystem
  stopwatch : stopwatch_ul/stopwatch  SystemSampleTime=-1  Latency=0  AutoFrameSizeCalculation=off
  lapNum : Outport  VectorParamsAs1DForOutWhenUnconnected=off
  rst : Outport  Port=2  VectorParamsAs1DForOutWhenUnconnected=off
  wires:
  Subsystem/1(realLap) -> Logical Operator1/3  "real"
  Compare To Constant1/1 -> Logical Operator1/4
  Memory/1 -> stopwatch/1, Subsystem/2(rst)
  stopwatch/1 -> Compare To Constant1/1
  pathParameter/1 -> Memory3/1, Compare To Constant3/1, Subsystem/1(S)
  Compare To Constant4/1 -> Logical Operator1/2
  Add2/1 -> Memory4/1, lapNum/1
  Memory4/1 -> Add2/2
  Logical Operator1/1 -> Memory/1, Data Type Conversion2/1, rst/1
  Data Type Conversion2/1 -> Add2/1
  Memory3/1 -> Compare To Constant4/1
  Compare To Constant3/1 -> Logical Operator1/1

== system MantaFSController_cl/MantaFSController/xcurrent-ellipse/pathFollowingControllerManta1/Subsystem ==
  posVecGnd : Inport
  Atan1 : Trigonometry  Operator=atan2
  Atan2 : Trigonometry  Operator=atan2
  Gain : Gain  Gain=180/pi
  Gain1 : Gain  Gain=180/pi
  Selector1 : Selector  InputPortWidth=3  IndexOptions=Index vector (dialog)  Indices=1  OutputSizes=1
  Selector2 : Selector  InputPortWidth=3  IndexOptions=Index vector (dialog)  Indices=[1 2]  OutputSizes=1
  Selector3 : Selector  InputPortWidth=3  IndexOptions=Index vector (dialog)  Indices=3  OutputSizes=1
  Selector4 : Selector  InputPortWidth=3  IndexOptions=Index vector (dialog)  Indices=2  OutputSizes=1
  Sqrt1 : Sqrt  SaturateOnIntegerOverflow=on
  Sqrt2 : Sqrt  SaturateOnIntegerOverflow=on
  Square1 : Math  Operator=square  SignedPower=on  SaturateOnIntegerOverflow=on
  Square2 : Math  Operator=square  SignedPower=on  SaturateOnIntegerOverflow=on
  Sum of Elements : Sum  Inputs=+
  Sum of Elements1 : Sum  Inputs=+
  elevationAngle : Outport
  azimuth Angle : Outport  Port=2
  wires:
  Gain1/1 -> azimuth Angle/1
  Selector4/1 -> Atan2/1
  Sqrt2/1 -> Atan2/2
  posVecGnd/1 -> Selector3/1, Selector2/1, Selector4/1, Selector1/1
  Selector1/1 -> Square2/1
  Sum of Elements1/1 -> Sqrt2/1
  Square2/1 -> Sum of Elements1/1
  Atan2/1 -> Gain1/1
  Gain/1 -> elevationAngle/1
  Selector2/1 -> Square1/1
  Atan1/1 -> Gain/1
  Sum of Elements/1 -> Sqrt1/1
  Selector3/1 -> Atan1/1
  Square1/1 -> Sum of Elements/1
  Sqrt1/1 -> Atan1/2

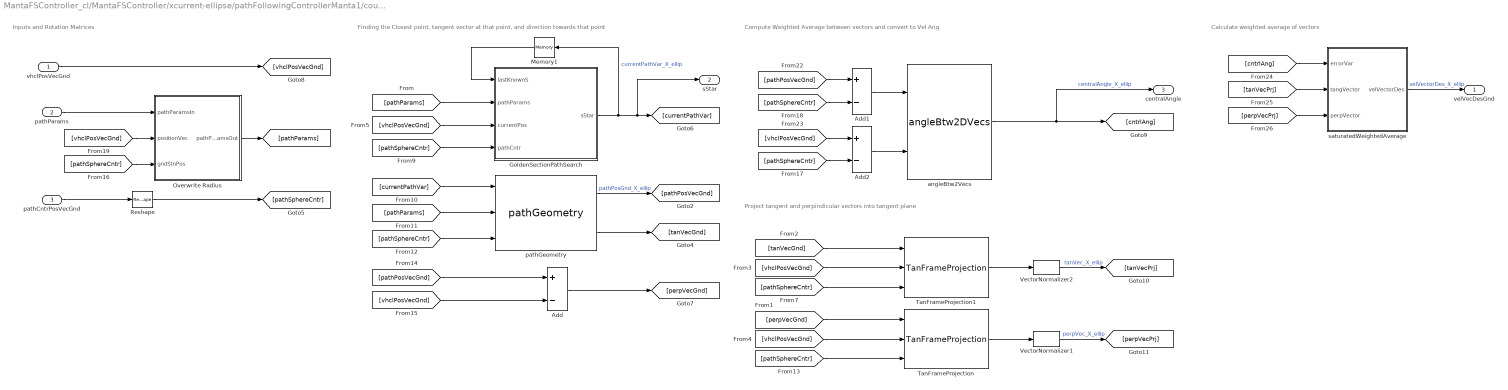
== system MantaFSController_cl/MantaFSController/xcurrent-ellipse/pathFollowingControllerManta1/courseFollowManta ==
  note: Finding the Closest point, tangent vector at that point, and direction towards that point
  note: Inputs and Rotation Matrices
  note: Compute Weighted Average between vectors and convert to Vel Ang
  note: Project tangent and perpindicular vectors into tangent plane
  note: Calculate weighted average of vectors
  "vhclPosVecGnd " : Inport
  pathParams : Inport  Port=2
  pathCntrPosVecGnd : Inport  Port=3
  Add : Sum  Inputs=+-
  Add1 : Sum  Inputs=+-
  Add2 : Sum  Inputs=+-
  GoldenSectionPathSearch : Subsystem  TreatAsAtomicUnit=on
  Memory1 : Memory  InitialCondition=pathCtrl.initPathVar.Value
  Overwrite Radius : Subsystem
  Reshape : Reshape  OutputDimensionality=Column vector (2-D)
  TanFrameProjection : tanFrameProjection_ul/TanFrameProjection  SystemSampleTime=-1  Latency=0  AutoFrameSizeCalculation=off
  TanFrameProjection1 : tanFrameProjection_ul/TanFrameProjection  SystemSampleTime=-1  Latency=0  AutoFrameSizeCalculation=off
  VectorNormalizer1 : vectorNormalizer_ul/VectorNormalizer   SystemSampleTime=-1  Latency=0  AutoFrameSizeCalculation=off
  VectorNormalizer2 : vectorNormalizer_ul/VectorNormalizer   SystemSampleTime=-1  Latency=0  AutoFrameSizeCalculation=off
  angleBtw2Vecs : angleBtw2Vecs_ul/angleBtw2DVecs  SystemSampleTime=-1  Latency=0  AutoFrameSizeCalculation=off
  pathGeometry : pathGeometry_ul/pathGeometry  SystemSampleTime=-1  Latency=0  AutoFrameSizeCalculation=off
  saturatedWeightedAverage : Subsystem  mask{error_upper_lim=pathCtrl.perpErrorVal.Value}
      mask prompts: error_upper_lim "Value of Error yielding 100% perpendicular"
  velVecDesGnd : Outport  VectorParamsAs1DForOutWhenUnconnected=off
  sStar : Outport  Port=2  VectorParamsAs1DForOutWhenUnconnected=off
  centralAngle : Outport  Port=3  VectorParamsAs1DForOutWhenUnconnected=off
  wires:
  saturatedWeightedAverage/1("velVectorDes ") -> velVecDesGnd/1  "velVectorDes_X_ellip"
  [perpVecPrj] -> saturatedWeightedAverage/3("perpVector ")
  [tanVecPrj] -> saturatedWeightedAverage/2(tangVector)
  [cntrlAng] -> saturatedWeightedAverage/1("errorVar ")
  [pathSphereCntr] -> TanFrameProjection/3
  [pathSphereCntr] -> TanFrameProjection1/3
  [vhclPosVecGnd] -> TanFrameProjection/2
  [vhclPosVecGnd] -> TanFrameProjection1/2
  [tanVecGnd] -> TanFrameProjection1/1
  [perpVecGnd] -> TanFrameProjection/1
  [vhclPosVecGnd] -> Overwrite Radius/2(positionVec)
  [pathSphereCntr] -> Overwrite Radius/3(gndStnPos)
  Add2/1 -> angleBtw2Vecs/2
  Add1/1 -> angleBtw2Vecs/1
  [pathSphereCntr] -> Add1/2
  [pathSphereCntr] -> Add2/2
  [pathSphereCntr] -> GoldenSectionPathSearch/4(pathCntr)
  [pathSphereCntr] -> pathGeometry/3
  Reshape/1 -> [pathSphereCntr]
  pathCntrPosVecGnd/1 -> Reshape/1
  Overwrite Radius/1(pathParamsOut) -> [pathParams]
  pathParams/1 -> Overwrite Radius/1(pathParamsIn)
  TanFrameProjection/1 -> VectorNormalizer1/1
  pathGeometry/2 -> [tanVecGnd]
  [pathPosVecGnd] -> Add/1
  [vhclPosVecGnd] -> Add/2
  Add/1 -> [perpVecGnd]
  Memory1/1 -> GoldenSectionPathSearch/1(lastKnownS)
  GoldenSectionPathSearch/1(sStar) -> [currentPathVar], sStar/1, Memory1/1  "currentPathVar_X_ellip"
  [pathParams] -> GoldenSectionPathSearch/2(pathParams)
  TanFrameProjection1/1 -> VectorNormalizer2/1
  [currentPathVar] -> pathGeometry/1
  [vhclPosVecGnd] -> Add2/1
  angleBtw2Vecs/1 -> centralAngle/1, [cntrlAng]  "centralAngle_X_ellip"
  VectorNormalizer1/1 -> [perpVecPrj]  "perpVec_X_ellip"
  [pathParams] -> pathGeometry/2
  pathGeometry/1 -> [pathPosVecGnd]  "pathPosGnd_X_ellip"
  "vhclPosVecGnd "/1 -> [vhclPosVecGnd]
  [vhclPosVecGnd] -> GoldenSectionPathSearch/3(currentPos)
  VectorNormalizer2/1 -> [tanVecPrj]  "tanVec_X_ellip"
  [pathPosVecGnd] -> Add1/1

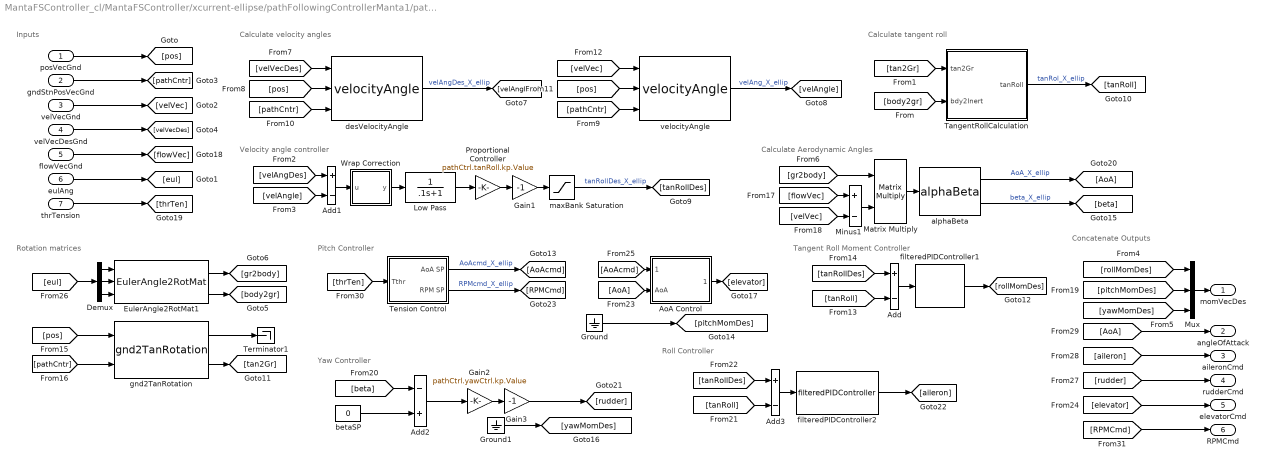
== system MantaFSController_cl/MantaFSController/xcurrent-ellipse/pathFollowingControllerManta1/pathTrackingCtrl ==
  note: Pitch Controller
  note: Calculate Aerodynamic Angles
  note: Yaw Controller
  note: Concatenate Outputs
  note: Tangent Roll Moment Controller
  note: Calculate tangent roll
  note: Calculate velocity angles
  note: Rotation matrices
  note: Inputs
  note: Velocity angle controller
  note: Roll Controller
  posVecGnd : Inport
  gndStnPosVecGnd : Inport  Port=2
  velVecGnd : Inport  Port=3
  velVecDesGnd : Inport  Port=4
  flowVecGnd : Inport  Port=5
  eulAng : Inport  Port=6
  thrTension : Inport  Port=7
  Add : Sum  Inputs=+-
  Add1 : Sum  Inputs=+-
  Add2 : Sum  Inputs=-+
  Add3 : Sum  Inputs=+-
  AoA Control : Subsystem
  Demux : Demux  Outputs=3
  EulerAngle2RotMat1 : eulAng2RotMat_ul/EulerAngle2RotMat  SystemSampleTime=-1  Latency=0  AutoFrameSizeCalculation=off
  Gain1 : Gain  Gain=-1
  Gain2 : Gain  Gain=pathCtrl.yawCtrl.kp.Value
  Gain3 : Gain  Gain=-1
  Ground : Ground
  Ground1 : Ground
  Low Pass : TransferFcn  Denominator=[.1 1]
  Matrix Multiply : Product  Multiplication=Matrix(*)
  Minus1 : Sum  Inputs=+-
  Mux : Mux  Inputs=3
  Proportional Controller : Gain  Gain=pathCtrl.tanRoll.kp.Value
  TangentRollCalculation : Subsystem
  Tension Control : Subsystem
  Terminator1 : Terminator
  Wrap Correction : Subsystem
  alphaBeta : alphaBeta_ul/alphaBeta  SystemSampleTime=-1  Latency=0  AutoFrameSizeCalculation=off
  betaSP : Constant  Value=0
  desVelocityAngle : velocityAngle_ul/velocityAngle  SystemSampleTime=-1  Latency=0  AutoFrameSizeCalculation=off
  filteredPIDController1 : filteredPIDController_ul/filteredPIDController  kp=pathCtrl.rollMoment.kp.Value  ki=0  kd=pathCtrl.rollMoment.kd.Value  Value=pathCtrl.rollMoment.tau.Value  externalReset=none
  filteredPIDController2 : filteredPIDController_ul/filteredPIDController  kp=pathCtrl.rollCtrl.kp.Value  ki=pathCtrl.rollCtrl.ki.Value  kd=pathCtrl.rollCtrl.kd.Value  Value=pathCtrl.rollCtrl.tau.Value  externalReset=none
  gnd2TanRotation : gnd2TanRotation_ul/gnd2TanRotation  SystemSampleTime=-1  Latency=0  AutoFrameSizeCalculation=off
  maxBank Saturation : Saturate  UpperLimit=pathCtrl.maxBank.upperLimit.Value  LowerLimit=pathCtrl.maxBank.lowerLimit.Value
  velocityAngle : velocityAngle_ul/velocityAngle  SystemSampleTime=-1  Latency=0  AutoFrameSizeCalculation=off
  momVecDes : Outport  VectorParamsAs1DForOutWhenUnconnected=off
  angleOfAttack : Outport  Port=2  VectorParamsAs1DForOutWhenUnconnected=off
  aileronCmd : Outport  Port=3  VectorParamsAs1DForOutWhenUnconnected=off
  rudderCmd : Outport  Port=4  VectorParamsAs1DForOutWhenUnconnected=off
  elevatorCmd : Outport  Port=5  VectorParamsAs1DForOutWhenUnconnected=off
  RPMCmd : Outport  Port=6  VectorParamsAs1DForOutWhenUnconnected=off
  wires:
  Ground1/1 -> [yawMomDes]
  Low Pass/1 -> Proportional Controller/1
  Wrap Correction/1(y) -> Low Pass/1
  Ground/1 -> [pitchMomDes]
  posVecGnd/1 -> [pos]
  velVecGnd/1 -> [velVec]
  Add/1 -> filteredPIDController1/1
  Proportional Controller/1 -> Gain1/1
  Gain1/1 -> maxBank Saturation/1
  maxBank Saturation/1 -> [tanRollDes]  "tanRollDes_X_ellip"
  Add1/1 -> Wrap Correction/1(u)
  flowVecGnd/1 -> [flowVec]
  [tan2Gr] -> TangentRollCalculation/1(tan2Gr)
  TangentRollCalculation/1(tanRoll) -> [tanRoll]  "tanRol_X_ellip"
  filteredPIDController1/1 -> [rollMomDes]
  Gain2/1 -> Gain3/1
  Minus1/1 -> Matrix Multiply/2
  [velVec] -> Minus1/2
  [flowVec] -> Minus1/1
  Demux/3 -> EulerAngle2RotMat1/3
  Demux/1 -> EulerAngle2RotMat1/1
  Demux/2 -> EulerAngle2RotMat1/2
  EulerAngle2RotMat1/2 -> [body2gr]
  EulerAngle2RotMat1/1 -> [gr2body]
  [body2gr] -> TangentRollCalculation/2(bdy2Inert)
  [gr2body] -> Matrix Multiply/1
  Matrix Multiply/1 -> alphaBeta/1
  alphaBeta/2 -> [beta]  "beta_X_ellip"
  Add2/1 -> Gain2/1
  Mux/1 -> momVecDes/1
  [pitchMomDes] -> Mux/2
  gndStnPosVecGnd/1 -> [pathCntr]
  velVecDesGnd/1 -> [velVecDes]
  desVelocityAngle/1 -> [velAngDes]  "velAngDes_X_ellip"
  velocityAngle/1 -> [velAngle]  "velAng_X_ellip"
  [velAngDes] -> Add1/1
  [velAngle] -> Add1/2
  [velVecDes] -> desVelocityAngle/1
  [pos] -> desVelocityAngle/2
  [pathCntr] -> desVelocityAngle/3
  [velVec] -> velocityAngle/1
  [tanRoll] -> Add/2
  [tanRollDes] -> Add/1
  [pos] -> gnd2TanRotation/1
  [pathCntr] -> gnd2TanRotation/2
  gnd2TanRotation/2 -> [tan2Gr]
  gnd2TanRotation/1 -> Terminator1/1
  [rollMomDes] -> Mux/1
  [yawMomDes] -> Mux/3
  Tension Control/2(RPM SP) -> [RPMCmd]  "RPMcmd_X_ellip"
  AoA Control/1(elvCmd) -> [elevator]
  Tension Control/1(AoA SP) -> [AoAcmd]  "AoAcmd_X_ellip"
  [AoAcmd] -> AoA Control/1(AoA SP)
  [AoA] -> AoA Control/2(AoA)
  eulAng/1 -> [eul]
  thrTension/1 -> [thrTen]
  [eul] -> Demux/1
  [thrTen] -> Tension Control/1(Tthr)
  [pos] -> velocityAngle/2
  [pathCntr] -> velocityAngle/3
  alphaBeta/1 -> [AoA]  "AoA_X_ellip"
  Gain3/1 -> [rudder]
  [beta] -> Add2/1
  betaSP/1 -> Add2/2
  filteredPIDController2/1 -> [aileron]
  [AoA] -> angleOfAttack/1
  [aileron] -> aileronCmd/1
  [rudder] -> rudderCmd/1
  [elevator] -> elevatorCmd/1
  [tanRollDes] -> Add3/1
  [tanRoll] -> Add3/2
  Add3/1 -> filteredPIDController2/1
  [RPMCmd] -> RPMCmd/1

== system MantaFSController_cl/MantaFSController/xcurrent-lemOfBooth/pathFollowingControllerManta/Concatenation ==
  In1 : Inport
  Demux1 : Demux
  Gain : Gain  Gain=pathCtrl.rudderGain.Value
  Mux : Mux
  Out1 : Outport
  wires:
  In1/1 -> Demux1/1
  Mux/1 -> Out1/1
  Demux1/4 -> Gain/1
  Gain/1 -> Mux/4  "rudderCmd"
  Demux1/2 -> Mux/2  "starBrdCmd"
  Demux1/1 -> Mux/1  "portCmd"
  Demux1/3 -> Mux/3  "elevCmd"
